simulink model "quad_1_ref_NN_ports_R2016a"  (R2016a)
settings: Solver=FixedStepAuto  SolverMode=SingleTasking  StartTime=0.0  StopTime=20  FixedStep=0.01  RelTol=1e-3
libraries: neural x416, simulink x2
(part 9 of 15)

== system quad_1_ref_NN_ports_R2016a/nn_2/Layer 3/Delays 1 ==
  "p{3}" : Inport  PortDimensions=30
      mask Display: e = 0.06;c1 = [120 230 180]/255;c2 = ([120 230 180]+0)/(256+128);c3 = ([120 230 180]+128)/(256+128);patch([0 1 1 0],[0 0 1 1],c1);patch([0 1 1 1-e 1-e 0+e],[0 0 1 1-e 0+e 0+e],c2);patch([0 0 1 1-e 0+e 0+e],[0 1 1 1-e 1-e 0+e],c3);plot([0 1 1 0 0],[0 0 1 1 0]);
  mux : Mux  Inputs=1
      mask Display: e = 0.06;c1 = [120 150 230]/255;c2 = ([120 150 230]+0)/383;c3 = ([120 150 230]+128)/383;patch([0 1 1 0],[0 0 1 1],c1);patch([0 1 1 1-e 1-e 0+e],[0 0 1 1-e 0+e 0+e],c2);patch([0 0 1 1-e 0+e 0+e],[0 1 1 1-e 1-e 0+e],c3);plot([0 1 1 0 0],[0 0 1 1 0]);disp('Mux')
  "pd{3,2}" : Outport
      mask Display: e = 0.06;c1 = [120 230 180]/255;c2 = ([120 230 180]+0)/(256+128);c3 = ([120 230 180]+128)/(256+128);patch([0 1 1 0],[0 0 1 1],c1);patch([0 1 1 1-e 1-e 0+e],[0 0 1 1-e 0+e 0+e],c2);patch([0 0 1 1-e 0+e 0+e],[0 1 1 1-e 1-e 0+e],c3);plot([0 1 1 0 0],[0 0 1 1 0]);
  wires:
  "p{3}"/1 -> mux/1
  mux/1 -> "pd{3,2}"/1

== system quad_1_ref_NN_ports_R2016a/nn_2/Layer 3/LW{3,2} ==
  "ad{3,2}" : Inport  PortDimensions=30
      mask Display: e = 0.06;c1 = [120 230 180]/255;c2 = ([120 230 180]+0)/(256+128);c3 = ([120 230 180]+128)/(256+128);patch([0 1 1 0],[0 0 1 1],c1);patch([0 1 1 1-e 1-e 0+e],[0 0 1 1-e 0+e 0+e],c2);patch([0 0 1 1-e 0+e 0+e],[0 1 1 1-e 1-e 0+e],c3);plot([0 1 1 0 0],[0 0 1 1 0]);
  "IW{3,2}(1,:)'" : Constant  Value=[-0.27926346020130399239178586867637932300567626953125;0.346606766393038834284112681416445411741733551025390625;-0.40463771690971828132177279258030466735363006591796875;0.374237250338739446675617728033103048801422119140625;0.253674479943673480963894917294965125620365142822265625;0.0770967057085971962937520629566279239952564239501953125;-0.202899235421085510910899074588087387382984161376953125;0.048789096197364538454177562698532710783183574676513671875;0.1969315529635952966014400544736417941749095916748046875;-0.22194913799231852369331363661331124603748321533203125;-0.10977738597411164367390057350348797626793384552001953125;-0.358002132240892556591660422782297246158123016357421875;-0.1503757586855622718768898948837886564433574676513671875;0.200219880617318768400991757516749203205108642578125;-0.123543856037150845406102916967938654124736785888671875;-0.0756290226239554608245185818304889835417270660400390625;0.09365695161798102963413015231708413921296596527099609375;-0.20471536813625856865428431774489581584930419921875;0.2120496832146524790463359977366053499281406402587890625;-0.372640774432040966512857949055614881217479705810546875;-0.0302653179057935893536690485916551551781594753265380859375;0.26262527413470404535900115661206655204296112060546875;0.135112314967465174664340565868769772350788116455078125;0.06986865315379715835053531236553681083023548126220703125;0.1380766631074236416854006392895826138556003570556640625;0.12643817431793713534915468699182383716106414794921875;-0.0841054694251663903514781850390136241912841796875;0.0107954259001523632244268213753457530401647090911865234375;-0.3098502314874116425613692626939155161380767822265625;-0.414602245804907398873950796769349835813045501708984375]
      mask Display: e = 0.06;c1 = [120 150 230]/255;c2 = ([120 150 230]+0)/383;c3 = ([120 150 230]+128)/383;patch([0 1 1 0],[0 0 1 1],c1);patch([0 1 1 1-e 1-e 0+e],[0 0 1 1-e 0+e 0+e],c2);patch([0 0 1 1-e 0+e 0+e],[0 1 1 1-e 1-e 0+e],c3);plot([0 1 1 0 0],[0 0 1 1 0]);disp('weights');
  "IW{3,2}(2,:)'" : Constant  Value=[-0.05747200023448355288291367060082848183810710906982421875;-0.0259577833702099060320112045019413926638662815093994140625;-0.0236994303769792295788487734853333677165210247039794921875;-0.031656006151221056932332231781401787884533405303955078125;0.02922803437695457862144365890344488434493541717529296875;-0.0138028700105828072697278230407391674816608428955078125;0.03581160208022715618625397837604396045207977294921875;0.112598189160304007483404120648629032075405120849609375;0.0278682772623776060794131836928499978967010974884033203125;0.01299548234236705922250987299548796727322041988372802734375;-0.0042449449882556132551680860842679976485669612884521484375;-0.0026716794761836083239858741222860771813429892063140869140625;-0.07927304809738729141077584472441230900585651397705078125;-0.0169222274978570695613822039149454212747514247894287109375;0.01453554486356052090345603033938459702767431735992431640625;0.0215353596980647384040441494335027527995407581329345703125;-0.04032680291918665227424156682900502346456050872802734375;-0.0759479482050604282061812000392819754779338836669921875;-0.006611013865375271227053932676653857924975454807281494140625;0.0031452949687314217704081631410417685401625931262969970703125;0.055297610322103320223963152102442109026014804840087890625;0.06198230119153878836524285134146339260041713714599609375;-0.0644313380485042885847946081412374041974544525146484375;-0.064363247549387880841464948389329947531223297119140625;-0.07785031888928649335124276831265888176858425140380859375;0.08416766991241975137683084540185518562793731689453125;0.0494813713765498708330170529734459705650806427001953125;-0.080233821303533348068270925068645738065242767333984375;-0.053953159457228984374754787722849869169294834136962890625;0.00844389404800993843835943408748789806850254535675048828125]
      mask Display: e = 0.06;c1 = [120 150 230]/255;c2 = ([120 150 230]+0)/383;c3 = ([120 150 230]+128)/383;patch([0 1 1 0],[0 0 1 1],c1);patch([0 1 1 1-e 1-e 0+e],[0 0 1 1-e 0+e 0+e],c2);patch([0 0 1 1-e 0+e 0+e],[0 1 1 1-e 1-e 0+e],c3);plot([0 1 1 0 0],[0 0 1 1 0]);disp('weights');
  "IW{3,2}(3,:)'" : Constant  Value=[-0.017218098925270992893832300296708126552402973175048828125;0.064559652034786141339139931005774997174739837646484375;-0.027977779266303494376533222975922399200499057769775390625;-0.01321248185154027567078660609922735602594912052154541015625;-0.0830621278421327657870421035113395191729068756103515625;-0.0010825688028150916471237241722747057792730629444122314453125;0.04702127339298324548710894532632664777338504791259765625;0.03579689634253153951437553814685088582336902618408203125;0.0722733893767697754828560618989286012947559356689453125;-0.001674565279581757305804590174602708430029451847076416015625;0.053646957375234116671691708688740618526935577392578125;0.07916322856407694008584741141021368093788623809814453125;-0.0129246026132422663079690750009831390343606472015380859375;0.059649020929645669986118861061186180450022220611572265625;-0.019698735030489515629437136112755979411303997039794921875;-0.052245577874222605407883435191251919604837894439697265625;-0.03210867066066773467536421549084479920566082000732421875;0.005740737672801155162816133525893746991641819477081298828125;-0.00965489046477303360094257556056618341244757175445556640625;-0.047030004358195674762921356659717275761067867279052734375;-0.03725889805072464533441944922742550261318683624267578125;0.052107784180737082291301476288936100900173187255859375;-0.060045653206628225861951619890533038415014743804931640625;-0.1206224460907344975257871055873692966997623443603515625;-0.00701652679878371487998123257057159207761287689208984375;0.1050073098366831880756677719546132721006870269775390625;-0.01056686890756637804689166415528234210796654224395751953125;-0.1311364635573339099128276075134635902941226959228515625;-0.054499355693794680755015491513404413126409053802490234375;0.05349236857790563848258358348175534047186374664306640625]
      mask Display: e = 0.06;c1 = [120 150 230]/255;c2 = ([120 150 230]+0)/383;c3 = ([120 150 230]+128)/383;patch([0 1 1 0],[0 0 1 1],c1);patch([0 1 1 1-e 1-e 0+e],[0 0 1 1-e 0+e 0+e],c2);patch([0 0 1 1-e 0+e 0+e],[0 1 1 1-e 1-e 0+e],c3);plot([0 1 1 0 0],[0 0 1 1 0]);disp('weights');
  Mux : Mux  Inputs=3
      mask Display: e = 0.06;c1 = [120 150 230]/255;c2 = ([120 150 230]+0)/383;c3 = ([120 150 230]+128)/383;patch([0 1 1 0],[0 0 1 1],c1);patch([0 1 1 1-e 1-e 0+e],[0 0 1 1-e 0+e 0+e],c2);patch([0 0 1 1-e 0+e 0+e],[0 1 1 1-e 1-e 0+e],c3);plot([0 1 1 0 0],[0 0 1 1 0]);disp('Mux');
  dotprod1 : neural/Weight Functions/dotprod
  dotprod2 : neural/Weight Functions/dotprod
  dotprod3 : neural/Weight Functions/dotprod
  "lz{3,2}" : Outport
      mask Display: e = 0.06;c1 = [120 230 180]/255;c2 = ([120 230 180]+0)/(256+128);c3 = ([120 230 180]+128)/(256+128);patch([0 1 1 0],[0 0 1 1],c1);patch([0 1 1 1-e 1-e 0+e],[0 0 1 1-e 0+e 0+e],c2);patch([0 0 1 1-e 0+e 0+e],[0 1 1 1-e 1-e 0+e],c3);plot([0 1 1 0 0],[0 0 1 1 0]);
  wires:
  "IW{3,2}(1,:)'"/1 -> dotprod1/1
  "ad{3,2}"/1 -> dotprod1/2, dotprod2/2, dotprod3/2
  dotprod1/1 -> Mux/1
  "IW{3,2}(2,:)'"/1 -> dotprod2/1
  dotprod2/1 -> Mux/2
  "IW{3,2}(3,:)'"/1 -> dotprod3/1
  dotprod3/1 -> Mux/3
  Mux/1 -> "lz{3,2}"/1

== system quad_1_ref_NN_ports_R2016a/nn_3_const/Layer 1/Delays 1 ==
  "p{1}" : Inport  PortDimensions=12
      mask Display: e = 0.06;c1 = [120 230 180]/255;c2 = ([120 230 180]+0)/(256+128);c3 = ([120 230 180]+128)/(256+128);patch([0 1 1 0],[0 0 1 1],c1);patch([0 1 1 1-e 1-e 0+e],[0 0 1 1-e 0+e 0+e],c2);patch([0 0 1 1-e 0+e 0+e],[0 1 1 1-e 1-e 0+e],c3);plot([0 1 1 0 0],[0 0 1 1 0]);
  mux : Mux  Inputs=1
      mask Display: e = 0.06;c1 = [120 150 230]/255;c2 = ([120 150 230]+0)/383;c3 = ([120 150 230]+128)/383;patch([0 1 1 0],[0 0 1 1],c1);patch([0 1 1 1-e 1-e 0+e],[0 0 1 1-e 0+e 0+e],c2);patch([0 0 1 1-e 0+e 0+e],[0 1 1 1-e 1-e 0+e],c3);plot([0 1 1 0 0],[0 0 1 1 0]);disp('Mux')
  "pd{1,1}" : Outport
      mask Display: e = 0.06;c1 = [120 230 180]/255;c2 = ([120 230 180]+0)/(256+128);c3 = ([120 230 180]+128)/(256+128);patch([0 1 1 0],[0 0 1 1],c1);patch([0 1 1 1-e 1-e 0+e],[0 0 1 1-e 0+e 0+e],c2);patch([0 0 1 1-e 0+e 0+e],[0 1 1 1-e 1-e 0+e],c3);plot([0 1 1 0 0],[0 0 1 1 0]);
  wires:
  "p{1}"/1 -> mux/1
  mux/1 -> "pd{1,1}"/1

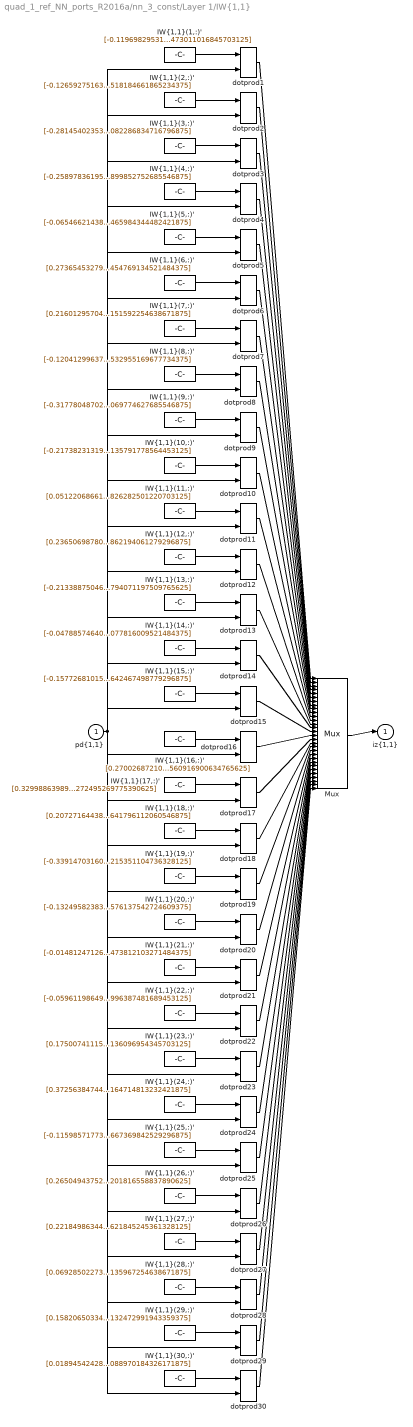
== system quad_1_ref_NN_ports_R2016a/nn_3_const/Layer 1/IW{1,1} ==
  "pd{1,1}" : Inport  PortDimensions=12
      mask Display: e = 0.06;c1 = [120 230 180]/255;c2 = ([120 230 180]+0)/(256+128);c3 = ([120 230 180]+128)/(256+128);patch([0 1 1 0],[0 0 1 1],c1);patch([0 1 1 1-e 1-e 0+e],[0 0 1 1-e 0+e 0+e],c2);patch([0 0 1 1-e 0+e 0+e],[0 1 1 1-e 1-e 0+e],c3);plot([0 1 1 0 0],[0 0 1 1 0]);
  "IW{1,1}(1,:)'" : Constant  Value=[-0.1196982953119827275401121369213797152042388916015625;-0.1289870733556734150315747911008656956255435943603515625;0.01486838419769767431766194221154364640824496746063232421875;-0.1972668416460273965729044221006915904581546783447265625;-0.1706947324630785356447404410573653876781463623046875;0.15527943735119176249526162791880778968334197998046875;0.280496872652939932546445334082818590104579925537109375;0.159230402032687179403325217208475805819034576416015625;-0.030182451792157276304617852247247355990111827850341796875;-0.09238192960821522969894203924923203885555267333984375;-0.09747367045827955156500621569648501463234424591064453125;0.1882049887453905168133161396326613612473011016845703125]
      mask Display: e = 0.06;c1 = [120 150 230]/255;c2 = ([120 150 230]+0)/383;c3 = ([120 150 230]+128)/383;patch([0 1 1 0],[0 0 1 1],c1);patch([0 1 1 1-e 1-e 0+e],[0 0 1 1-e 0+e 0+e],c2);patch([0 0 1 1-e 0+e 0+e],[0 1 1 1-e 1-e 0+e],c3);plot([0 1 1 0 0],[0 0 1 1 0]);disp('Weights');
  "IW{1,1}(10,:)'" : Constant  Value=[-0.2173823131999155500171383437191252596676349639892578125;-0.25150582247166453075948311379761435091495513916015625;-0.22407324408224360556829424240277148783206939697265625;-0.0178235762451871282419091357951401732861995697021484375;-0.0857934106951768471471808652495383284986019134521484375;0.19276250346259404810922433171072043478488922119140625;0.09913209349963171546082918439424247480928897857666015625;-0.0588047207570860652747768426706898026168346405029296875;-0.09416480925285675152025532952393405139446258544921875;0.1629371022116075373720178731673513539135456085205078125;-0.1852160572554303608061587738120579160749912261962890625;0.1669185592333850554069840654847212135791778564453125]
      mask Display: e = 0.06;c1 = [120 150 230]/255;c2 = ([120 150 230]+0)/383;c3 = ([120 150 230]+128)/383;patch([0 1 1 0],[0 0 1 1],c1);patch([0 1 1 1-e 1-e 0+e],[0 0 1 1-e 0+e 0+e],c2);patch([0 0 1 1-e 0+e 0+e],[0 1 1 1-e 1-e 0+e],c3);plot([0 1 1 0 0],[0 0 1 1 0]);disp('Weights');
  "IW{1,1}(11,:)'" : Constant  Value=[0.0512206866191046439329426220865570940077304840087890625;-0.1510948101597614223745580375179997645318508148193359375;-0.2129182130455107568867134659740258939564228057861328125;-0.342260556306487939703941947300336323678493499755859375;0.09978610256588016369505567126907408237457275390625;0.08653903693296537136259161115958704613149166107177734375;0.0034675135718981284389805797019334931974299252033233642578125;-0.178171083527447093874940264868200756609439849853515625;0.1926456653787382011788764657467254437506198883056640625;-0.2155749799301446556487604766516597010195255279541015625;-0.09451893403511162083940888578581507317721843719482421875;-0.04709443449216606236706894605958950705826282501220703125]
      mask Display: e = 0.06;c1 = [120 150 230]/255;c2 = ([120 150 230]+0)/383;c3 = ([120 150 230]+128)/383;patch([0 1 1 0],[0 0 1 1],c1);patch([0 1 1 1-e 1-e 0+e],[0 0 1 1-e 0+e 0+e],c2);patch([0 0 1 1-e 0+e 0+e],[0 1 1 1-e 1-e 0+e],c3);plot([0 1 1 0 0],[0 0 1 1 0]);disp('Weights');
  "IW{1,1}(12,:)'" : Constant  Value=[0.2365069878030960082160305546494782902300357818603515625;0.29432103747985538522158321939059533178806304931640625;0.2081499956215297764128280277873273007571697235107421875;0.25117398464888995857080544737982563674449920654296875;-0.2485034489625476961105476902957889251410961151123046875;0.158395104552063348268831077803042717278003692626953125;-0.1044569536603661419338351379337836988270282745361328125;-0.22613789129050088089201153707108460366725921630859375;-0.10573345075038453888538469982449896633625030517578125;0.02215455254487565250887115553268813528120517730712890625;0.027546109987116075557000982598765403963625431060791015625;-0.0492491638251608410126181070154416374862194061279296875]
      mask Display: e = 0.06;c1 = [120 150 230]/255;c2 = ([120 150 230]+0)/383;c3 = ([120 150 230]+128)/383;patch([0 1 1 0],[0 0 1 1],c1);patch([0 1 1 1-e 1-e 0+e],[0 0 1 1-e 0+e 0+e],c2);patch([0 0 1 1-e 0+e 0+e],[0 1 1 1-e 1-e 0+e],c3);plot([0 1 1 0 0],[0 0 1 1 0]);disp('Weights');
  "IW{1,1}(13,:)'" : Constant  Value=[-0.21338875046561300852232534452923573553562164306640625;-0.1340059789318859551077167679977719672024250030517578125;-0.1476616545504399746757684397380216978490352630615234375;0.214969424376130813225671545296791009604930877685546875;0.06644921596088482207420611302950419485569000244140625;-0.0117821724168989082348613095518885529600083827972412109375;-0.1872827624335566543134490302691119723021984100341796875;-0.082787703128192280388475410290993750095367431640625;0.1926407037939068256360286568451556377112865447998046875;0.277999477762065627661769440237549133598804473876953125;0.1379735123752584835532530860291444696485996246337890625;-0.1613026880844560528860398562756017781794071197509765625]
      mask Display: e = 0.06;c1 = [120 150 230]/255;c2 = ([120 150 230]+0)/383;c3 = ([120 150 230]+128)/383;patch([0 1 1 0],[0 0 1 1],c1);patch([0 1 1 1-e 1-e 0+e],[0 0 1 1-e 0+e 0+e],c2);patch([0 0 1 1-e 0+e 0+e],[0 1 1 1-e 1-e 0+e],c3);plot([0 1 1 0 0],[0 0 1 1 0]);disp('Weights');
  "IW{1,1}(14,:)'" : Constant  Value=[-0.04788574640253502601172641561788623221218585968017578125;0.15070670290952647984994428043137304484844207763671875;0.129709002988810606638026001746766269207000732421875;-0.07628835032242430036486524613792425952851772308349609375;-0.064693014780291324683503262349404394626617431640625;-0.120818118544549601978133068769238889217376708984375;-0.133195843769588317950791633847984485328197479248046875;-0.006931056317864360376279631026363858836703002452850341796875;0.07580874238176138479872179232188500463962554931640625;-0.1738726228089309266966466793746803887188434600830078125;0.08809580303368071130254435274764546193182468414306640625;-0.34741805583377372013131889616488479077816009521484375]
      mask Display: e = 0.06;c1 = [120 150 230]/255;c2 = ([120 150 230]+0)/383;c3 = ([120 150 230]+128)/383;patch([0 1 1 0],[0 0 1 1],c1);patch([0 1 1 1-e 1-e 0+e],[0 0 1 1-e 0+e 0+e],c2);patch([0 0 1 1-e 0+e 0+e],[0 1 1 1-e 1-e 0+e],c3);plot([0 1 1 0 0],[0 0 1 1 0]);disp('Weights');
  "IW{1,1}(15,:)'" : Constant  Value=[-0.1577268101593818083738796076431754045188426971435546875;-0.11256779664810658003748500277652055956423282623291015625;0.00802241259106954533730782230804834398441016674041748046875;0.19139711738853704137142131003201939165592193603515625;0.14056375245487162661817137632169760763645172119140625;0.169850393957305667580470753819099627435207366943359375;-0.162927276810809373852606540822307579219341278076171875;0.0411550400127098925384672156724263913929462432861328125;-0.09100914000223625510699321239371784031391143798828125;0.260212573300696636824369534224388189613819122314453125;0.2000730920156783276819822958714212290942668914794921875;0.211937407148370116072300106679904274642467498779296875]
      mask Display: e = 0.06;c1 = [120 150 230]/255;c2 = ([120 150 230]+0)/383;c3 = ([120 150 230]+128)/383;patch([0 1 1 0],[0 0 1 1],c1);patch([0 1 1 1-e 1-e 0+e],[0 0 1 1-e 0+e 0+e],c2);patch([0 0 1 1-e 0+e 0+e],[0 1 1 1-e 1-e 0+e],c3);plot([0 1 1 0 0],[0 0 1 1 0]);disp('Weights');
  "IW{1,1}(16,:)'" : Constant  Value=[0.27002687210488574010014417581260204315185546875;-0.04349468469703339501553074342155014164745807647705078125;0.1330845919116534492587788918172009289264678955078125;-0.182575685011664157197941449339850805699825286865234375;-0.10830309161015201635525073697863263078033924102783203125;0.239269603992316504115223096960107795894145965576171875;0.04760708347616089686216156451337155885994434356689453125;0.11252778570572473382238598560434184037148952484130859375;-0.1548024416375938516754473539549508132040500640869140625;-0.253057365838928294277110353505122475326061248779296875;-0.1250555668859235358691961437216377817094326019287109375;0.047842143321554821133734236582313315011560916900634765625]
      mask Display: e = 0.06;c1 = [120 150 230]/255;c2 = ([120 150 230]+0)/383;c3 = ([120 150 230]+128)/383;patch([0 1 1 0],[0 0 1 1],c1);patch([0 1 1 1-e 1-e 0+e],[0 0 1 1-e 0+e 0+e],c2);patch([0 0 1 1-e 0+e 0+e],[0 1 1 1-e 1-e 0+e],c3);plot([0 1 1 0 0],[0 0 1 1 0]);disp('Weights');
  "IW{1,1}(17,:)'" : Constant  Value=[0.3299886398943197018951423160615377128124237060546875;0.0808292241972947966832663269087788648903369903564453125;-0.02259926392819711082893263665027916431427001953125;0.054982407635770051690382587139538372866809368133544921875;-0.160980157363610765219874565445934422314167022705078125;0.1247636296345608908353597144014202058315277099609375;-0.035927420779184739141332016743035637773573398590087890625;0.08232447522588388910680379240147885866463184356689453125;-0.346576289182833063851063570837141014635562896728515625;-0.034377817283129170899957927076684427447617053985595703125;-0.2185372357072770943542394661562866531312465667724609375;-0.01525722862075677178916865983637762838043272495269775390625]
      mask Display: e = 0.06;c1 = [120 150 230]/255;c2 = ([120 150 230]+0)/383;c3 = ([120 150 230]+128)/383;patch([0 1 1 0],[0 0 1 1],c1);patch([0 1 1 1-e 1-e 0+e],[0 0 1 1-e 0+e 0+e],c2);patch([0 0 1 1-e 0+e 0+e],[0 1 1 1-e 1-e 0+e],c3);plot([0 1 1 0 0],[0 0 1 1 0]);disp('Weights');
  "IW{1,1}(18,:)'" : Constant  Value=[0.2072716443886149229047788367097382433712482452392578125;-0.158695591362616961195186604527407325804233551025390625;-0.194298743989455957592582535653491504490375518798828125;0.08089761317006245733285396681822021491825580596923828125;0.1275882176345632945668739921529777348041534423828125;0.166975404185521092426114364570821635425090789794921875;0.2179788041767063144771299221247318200767040252685546875;-0.2113613415917590943049475527004688046872615814208984375;-0.1680332296617765008850398089634836651384830474853515625;0.09479967011305796831255321421849657781422138214111328125;-0.10581935301708489394201251343474723398685455322265625;0.1349044775358076986293554000440053641796112060546875]
      mask Display: e = 0.06;c1 = [120 150 230]/255;c2 = ([120 150 230]+0)/383;c3 = ([120 150 230]+128)/383;patch([0 1 1 0],[0 0 1 1],c1);patch([0 1 1 1-e 1-e 0+e],[0 0 1 1-e 0+e 0+e],c2);patch([0 0 1 1-e 0+e 0+e],[0 1 1 1-e 1-e 0+e],c3);plot([0 1 1 0 0],[0 0 1 1 0]);disp('Weights');
  "IW{1,1}(19,:)'" : Constant  Value=[-0.33914703160923675984150804652017541229724884033203125;-0.10453048735648527711727950872955261729657649993896484375;-0.212564469375703168907421058975160121917724609375;0.10608477723513420887258007496711798012256622314453125;0.06988075897708780070960443708827369846403598785400390625;-0.028392761793704111850100701985866180621087551116943359375;0.036008968898993153062715322221265523694455623626708984375;-0.1601325327805253329049861577004776336252689361572265625;-0.016320432310186705482379920795210637152194976806640625;-0.22994571208807734752355145246838219463825225830078125;0.036023256587950823470745120857827714644372463226318359375;0.20727117665203309559984745646943338215351104736328125]
      mask Display: e = 0.06;c1 = [120 150 230]/255;c2 = ([120 150 230]+0)/383;c3 = ([120 150 230]+128)/383;patch([0 1 1 0],[0 0 1 1],c1);patch([0 1 1 1-e 1-e 0+e],[0 0 1 1-e 0+e 0+e],c2);patch([0 0 1 1-e 0+e 0+e],[0 1 1 1-e 1-e 0+e],c3);plot([0 1 1 0 0],[0 0 1 1 0]);disp('Weights');
  "IW{1,1}(2,:)'" : Constant  Value=[-0.1265927516381810391532525272850762121379375457763671875;-0.10406462981791535227227285531625966541469097137451171875;0.2148185548406552902722665976398275233805179595947265625;0.2371580895787383791439850710958126001060009002685546875;-0.2365432498183281662118560007002088241279125213623046875;0.05987656335314291144999998550702002830803394317626953125;0.0222476006243518854843532750464873970486223697662353515625;-0.11668078404641089862447955738389282487332820892333984375;-0.065758349599259913187410120372078381478786468505859375;-0.1329431588756458670896876128608710132539272308349609375;-0.1338080838789649507081236379235633648931980133056640625;0.1707220913756906932601253856773837469518184661865234375]
      mask Display: e = 0.06;c1 = [120 150 230]/255;c2 = ([120 150 230]+0)/383;c3 = ([120 150 230]+128)/383;patch([0 1 1 0],[0 0 1 1],c1);patch([0 1 1 1-e 1-e 0+e],[0 0 1 1-e 0+e 0+e],c2);patch([0 0 1 1-e 0+e 0+e],[0 1 1 1-e 1-e 0+e],c3);plot([0 1 1 0 0],[0 0 1 1 0]);disp('Weights');
  "IW{1,1}(20,:)'" : Constant  Value=[-0.13249582383027558307730942033231258392333984375;0.040030613773851704551010044497161288745701313018798828125;0.1702824726947762545847808723920024931430816650390625;-0.2408725064798178105984760577484848909080028533935546875;0.10623812004958511912011687172707752324640750885009765625;-0.139869975143498359582139300982817076146602630615234375;-0.1723200936692933227245561056406586430966854095458984375;-0.03984927795910563064207821071249782107770442962646484375;0.044199567930560519635196925491982256062328815460205078125;-0.2190396426762913628660811582449241541326045989990234375;0.1277829387419819051618929961477988399565219879150390625;0.170374810191310677165432707624859176576137542724609375]
      mask Display: e = 0.06;c1 = [120 150 230]/255;c2 = ([120 150 230]+0)/383;c3 = ([120 150 230]+128)/383;patch([0 1 1 0],[0 0 1 1],c1);patch([0 1 1 1-e 1-e 0+e],[0 0 1 1-e 0+e 0+e],c2);patch([0 0 1 1-e 0+e 0+e],[0 1 1 1-e 1-e 0+e],c3);plot([0 1 1 0 0],[0 0 1 1 0]);disp('Weights');
  "IW{1,1}(21,:)'" : Constant  Value=[-0.0148124712623549335821504513432955718599259853363037109375;-0.0311784914315909322812814252756652422249317169189453125;0.04522188239780784713151007281339843757450580596923828125;-0.2934434913415149281945559778250753879547119140625;0.171158930875923209757871745750890113413333892822265625;-0.1608476581751500933403775661645340733230113983154296875;-0.20675638704950161095297289648442529141902923583984375;0.348156303749445783513039032186497934162616729736328125;0.23679845860962200898569562923512421548366546630859375;0.223892726248125562005242272789473645389080047607421875;0.0289030250850557980657473677865709760226309299468994140625;-0.235499357660744423892396071096300147473812103271484375]
      mask Display: e = 0.06;c1 = [120 150 230]/255;c2 = ([120 150 230]+0)/383;c3 = ([120 150 230]+128)/383;patch([0 1 1 0],[0 0 1 1],c1);patch([0 1 1 1-e 1-e 0+e],[0 0 1 1-e 0+e 0+e],c2);patch([0 0 1 1-e 0+e 0+e],[0 1 1 1-e 1-e 0+e],c3);plot([0 1 1 0 0],[0 0 1 1 0]);disp('Weights');
  "IW{1,1}(22,:)'" : Constant  Value=[-0.059611986491373301910723370156119926832616329193115234375;0.2213751577076687737655191767771611921489238739013671875;0.1589485844453750740257191864657215774059295654296875;0.197716121842041570033643438364379107952117919921875;0.1514662645304741539487025647758855484426021575927734375;0.172775003422918349560433171063777990639209747314453125;0.203060971850576976738267376276780851185321807861328125;0.036534503618149305470552690167096443474292755126953125;0.077301466994075640482009248444228433072566986083984375;-0.1177192604996646074777544299649889580905437469482421875;0.12106019577847100532341784173695486970245838165283203125;-0.17993851102336766434319770269212312996387481689453125]
      mask Display: e = 0.06;c1 = [120 150 230]/255;c2 = ([120 150 230]+0)/383;c3 = ([120 150 230]+128)/383;patch([0 1 1 0],[0 0 1 1],c1);patch([0 1 1 1-e 1-e 0+e],[0 0 1 1-e 0+e 0+e],c2);patch([0 0 1 1-e 0+e 0+e],[0 1 1 1-e 1-e 0+e],c3);plot([0 1 1 0 0],[0 0 1 1 0]);disp('Weights');
  "IW{1,1}(23,:)'" : Constant  Value=[0.175007411157043712979231031567906029522418975830078125;-0.09330095053247415559649624583471450023353099822998046875;-0.215960552939064631683407924356288276612758636474609375;0.129472414805143209992621677884017117321491241455078125;-0.239940808198920496607797758770175278186798095703125;-0.069653398870320959446189590380527079105377197265625;-0.214353875622127210132106256423867307603359222412109375;0.0004286375228889800488400740885452933071064762771129608154296875;-0.0512173795049029878523327852235524915158748626708984375;0.11594052081714589785832458801451139152050018310546875;-0.1445651588249391716889391545919352211058139801025390625;-0.25233328001959531849962559135747142136096954345703125]
      mask Display: e = 0.06;c1 = [120 150 230]/255;c2 = ([120 150 230]+0)/383;c3 = ([120 150 230]+128)/383;patch([0 1 1 0],[0 0 1 1],c1);patch([0 1 1 1-e 1-e 0+e],[0 0 1 1-e 0+e 0+e],c2);patch([0 0 1 1-e 0+e 0+e],[0 1 1 1-e 1-e 0+e],c3);plot([0 1 1 0 0],[0 0 1 1 0]);disp('Weights');
  "IW{1,1}(24,:)'" : Constant  Value=[0.37256384744881809734096123065683059394359588623046875;-0.1432842251991764126461958994696033187210559844970703125;0.1377718344421794693932525888158124871551990509033203125;-0.589353589211446315943021545535884797573089599609375;-0.06178531294047295840954348022933118045330047607421875;-0.0154505347069833799678040264780065626837313175201416015625;0.1683078258323121578765579897662973962724208831787109375;-0.1664437272399152123458776486586430110037326812744140625;0.1873791777907282962711832396962563507258892059326171875;0.03288416218820687519919232499887584708631038665771484375;0.162765271872292782706637126466375775635242462158203125;-0.11285274050517050958841736019167001359164714813232421875]
      mask Display: e = 0.06;c1 = [120 150 230]/255;c2 = ([120 150 230]+0)/383;c3 = ([120 150 230]+128)/383;patch([0 1 1 0],[0 0 1 1],c1);patch([0 1 1 1-e 1-e 0+e],[0 0 1 1-e 0+e 0+e],c2);patch([0 0 1 1-e 0+e 0+e],[0 1 1 1-e 1-e 0+e],c3);plot([0 1 1 0 0],[0 0 1 1 0]);disp('Weights');
  "IW{1,1}(25,:)'" : Constant  Value=[-0.115985717734956583768735072226263582706451416015625;0.1493076208638430546482567251587170176208019256591796875;0.2002476867355400813597299247703631408512592315673828125;-0.26771207475659564156700298553914763033390045166015625;0.057630772409985257798137325835341471247375011444091796875;-0.1617184235669213432373680916498415172100067138671875;0.0887999943613410336329394567655981518328189849853515625;0.1870226133578477278884832912808633409440517425537109375;0.2072915270584706759482429561103344894945621490478515625;-0.1819923377068865255612450937405810691416263580322265625;-0.11884873510801842455553156696623773314058780670166015625;0.132748019518751536605094543119776062667369842529296875]
      mask Display: e = 0.06;c1 = [120 150 230]/255;c2 = ([120 150 230]+0)/383;c3 = ([120 150 230]+128)/383;patch([0 1 1 0],[0 0 1 1],c1);patch([0 1 1 1-e 1-e 0+e],[0 0 1 1-e 0+e 0+e],c2);patch([0 0 1 1-e 0+e 0+e],[0 1 1 1-e 1-e 0+e],c3);plot([0 1 1 0 0],[0 0 1 1 0]);disp('Weights');
  "IW{1,1}(26,:)'" : Constant  Value=[0.265049437520101960341634139695088379085063934326171875;-0.043127962986870327366517585687688551843166351318359375;0.06324231785530269600581476652223500423133373260498046875;-0.167145498219675392448380080168135464191436767578125;-0.10266957509710296359006775901434593833982944488525390625;0.07046395097403711227368461322839721105992794036865234375;-0.0400817962941015792921461979858577251434326171875;-0.120489126858635497985261508802068419754505157470703125;0.2112149275665802239387858207919634878635406494140625;0.1891994577758218387675270832914975471794605255126953125;-0.228634657789148099116260937080369330942630767822265625;-0.10414946107419044418751497005359851755201816558837890625]
      mask Display: e = 0.06;c1 = [120 150 230]/255;c2 = ([120 150 230]+0)/383;c3 = ([120 150 230]+128)/383;patch([0 1 1 0],[0 0 1 1],c1);patch([0 1 1 1-e 1-e 0+e],[0 0 1 1-e 0+e 0+e],c2);patch([0 0 1 1-e 0+e 0+e],[0 1 1 1-e 1-e 0+e],c3);plot([0 1 1 0 0],[0 0 1 1 0]);disp('Weights');
  "IW{1,1}(27,:)'" : Constant  Value=[0.2218498634465736751852915631388896144926548004150390625;-0.193833751064416082154906462164944969117641448974609375;0.177941926350075052543076026267954148352146148681640625;-0.189252378762839124082262287629419006407260894775390625;0.1302286515182972947979322952960501424968242645263671875;-0.08080312339151420053529051301666186191141605377197265625;0.190680986355462211978561981595703400671482086181640625;0.00784100937892250222926993075134305399842560291290283203125;-0.044533453815674979570093938718855497427284717559814453125;0.1226007069319831888076777204332756809890270233154296875;-0.143956039601102980807212361469282768666744232177734375;-0.1712952981268955898741523924400098621845245361328125]
      mask Display: e = 0.06;c1 = [120 150 230]/255;c2 = ([120 150 230]+0)/383;c3 = ([120 150 230]+128)/383;patch([0 1 1 0],[0 0 1 1],c1);patch([0 1 1 1-e 1-e 0+e],[0 0 1 1-e 0+e 0+e],c2);patch([0 0 1 1-e 0+e 0+e],[0 1 1 1-e 1-e 0+e],c3);plot([0 1 1 0 0],[0 0 1 1 0]);disp('Weights');
  "IW{1,1}(28,:)'" : Constant  Value=[0.069285022730961542958283416737685911357402801513671875;0.260500037412751350718309595322352834045886993408203125;0.258929936548664585416190675459802150726318359375;0.051862203376026420886812928756626206450164318084716796875;-0.268011929124568393234540053526870906352996826171875;-0.047632612230134978303919268682875554077327251434326171875;0.0213582840605084124663282096889815875329077243804931640625;-0.1722721696730589169277436667471192777156829833984375;-0.1408531121301170030424287915593595243990421295166015625;-0.061585673930256552843776063355107908137142658233642578125;0.21738059838316259320123435827554203569889068603515625;0.0870751102544260191518077363070915453135967254638671875]
      mask Display: e = 0.06;c1 = [120 150 230]/255;c2 = ([120 150 230]+0)/383;c3 = ([120 150 230]+128)/383;patch([0 1 1 0],[0 0 1 1],c1);patch([0 1 1 1-e 1-e 0+e],[0 0 1 1-e 0+e 0+e],c2);patch([0 0 1 1-e 0+e 0+e],[0 1 1 1-e 1-e 0+e],c3);plot([0 1 1 0 0],[0 0 1 1 0]);disp('Weights');
  "IW{1,1}(29,:)'" : Constant  Value=[0.158206503345123372650249393700505606830120086669921875;-0.1167115813229379350790537728244089521467685699462890625;-0.174624619944309167340890098785166628658771514892578125;0.118069241875576214084730963804759085178375244140625;0.0858192857803793673898695715251960791647434234619140625;0.1588419771976567751448072840503300540149211883544921875;0.11195652437048354832516139367726282216608524322509765625;-0.2078568334560400299171334381753695197403430938720703125;-0.1216025675984538645391097588799311779439449310302734375;0.1442203309680535061598760648848838172852993011474609375;-0.11457073589732448548605958649204694665968418121337890625;-0.2423468718021511703053505470961681567132472991943359375]
      mask Display: e = 0.06;c1 = [120 150 230]/255;c2 = ([120 150 230]+0)/383;c3 = ([120 150 230]+128)/383;patch([0 1 1 0],[0 0 1 1],c1);patch([0 1 1 1-e 1-e 0+e],[0 0 1 1-e 0+e 0+e],c2);patch([0 0 1 1-e 0+e 0+e],[0 1 1 1-e 1-e 0+e],c3);plot([0 1 1 0 0],[0 0 1 1 0]);disp('Weights');
  "IW{1,1}(3,:)'" : Constant  Value=[-0.28145402353184112431705443668761290609836578369140625;0.1260781948537200436444294382454245351254940032958984375;-0.141407770914534658412975431929226033389568328857421875;0.0823049572737721835125057623372413218021392822265625;-0.2050827811065634997955697826910181902348995208740234375;0.1652183450870099712393113122743670828640460968017578125;-0.147211741015504105067890350255765952169895172119140625;0.273411467720603928999167919755564071238040924072265625;0.1614958034400274800024277510601677931845188140869140625;-0.03454812947097267439300338764951447956264019012451171875;-0.05152166018603630825989370123352273367345333099365234375;-0.025257365527026613694072665339263039641082286834716796875]
      mask Display: e = 0.06;c1 = [120 150 230]/255;c2 = ([120 150 230]+0)/383;c3 = ([120 150 230]+128)/383;patch([0 1 1 0],[0 0 1 1],c1);patch([0 1 1 1-e 1-e 0+e],[0 0 1 1-e 0+e 0+e],c2);patch([0 0 1 1-e 0+e 0+e],[0 1 1 1-e 1-e 0+e],c3);plot([0 1 1 0 0],[0 0 1 1 0]);disp('Weights');
  "IW{1,1}(30,:)'" : Constant  Value=[0.018945424280687926665844855733666918240487575531005859375;0.1995715801428248614701743690602597780525684356689453125;0.12403009923170328632213710307041765190660953521728515625;-0.06135912715795650840266972636527498252689838409423828125;-0.032326994868567771046485859187669120728969573974609375;-0.1798706547556056245529276793604367412626743316650390625;-0.0160351695508717702332024401812304859049618244171142578125;-0.083546644247350254630646304576657712459564208984375;-0.1951457803110835664828215385568910278379917144775390625;-0.1691544971538902208951782313306466676294803619384765625;-0.2066097784601954867600426268836599774658679962158203125;-0.2325971246851534501853819847383419983088970184326171875]
      mask Display: e = 0.06;c1 = [120 150 230]/255;c2 = ([120 150 230]+0)/383;c3 = ([120 150 230]+128)/383;patch([0 1 1 0],[0 0 1 1],c1);patch([0 1 1 1-e 1-e 0+e],[0 0 1 1-e 0+e 0+e],c2);patch([0 0 1 1-e 0+e 0+e],[0 1 1 1-e 1-e 0+e],c3);plot([0 1 1 0 0],[0 0 1 1 0]);disp('Weights');
  "IW{1,1}(4,:)'" : Constant  Value=[-0.25897836195603141096199806270305998623371124267578125;-0.08773584389797840776825665898286388255655765533447265625;0.12015507045280286735344787985013681463897228240966796875;0.0361909909585266531539815559881390072405338287353515625;-0.2128536070269596847115423088325769640505313873291015625;0.1463695284926984918616454933726345188915729522705078125;0.30953078911182541066438034249586053192615509033203125;-0.2034985363635319621788966060194070450961589813232421875;-0.0885619727404492185218742861252394504845142364501953125;-0.05643587643771015571747540207070414908230304718017578125;-0.2063731608513614534938795941343414597213268280029296875;0.1133056984907023501119027741879108361899852752685546875]
      mask Display: e = 0.06;c1 = [120 150 230]/255;c2 = ([120 150 230]+0)/383;c3 = ([120 150 230]+128)/383;patch([0 1 1 0],[0 0 1 1],c1);patch([0 1 1 1-e 1-e 0+e],[0 0 1 1-e 0+e 0+e],c2);patch([0 0 1 1-e 0+e 0+e],[0 1 1 1-e 1-e 0+e],c3);plot([0 1 1 0 0],[0 0 1 1 0]);disp('Weights');
  "IW{1,1}(5,:)'" : Constant  Value=[-0.06546621438372472734368301416907343082129955291748046875;-0.1405605935952531637678220022280584089457988739013671875;-0.224987235141161701079681733972392976284027099609375;0.2334506280952731993583171288264566101133823394775390625;0.062248364259608467141671184208462364040315151214599609375;0.2226942814012638771625773870255216024816036224365234375;0.1768548726666858972311757725037750788033008575439453125;0.05880562753752312243893385357296210713684558868408203125;-0.002704041070264113881538303729712424683384597301483154296875;0.192654298910743093653508140050689689815044403076171875;-0.1480341744715330254411611576870200224220752716064453125;-0.002533840567329140140706567052575337584130465984344482421875]
      mask Display: e = 0.06;c1 = [120 150 230]/255;c2 = ([120 150 230]+0)/383;c3 = ([120 150 230]+128)/383;patch([0 1 1 0],[0 0 1 1],c1);patch([0 1 1 1-e 1-e 0+e],[0 0 1 1-e 0+e 0+e],c2);patch([0 0 1 1-e 0+e 0+e],[0 1 1 1-e 1-e 0+e],c3);plot([0 1 1 0 0],[0 0 1 1 0]);disp('Weights');
  "IW{1,1}(6,:)'" : Constant  Value=[0.27365453279568419109324395321891643106937408447265625;0.197726059436817258596619240051950328052043914794921875;-0.0072955368385953338339344753649129415862262248992919921875;-0.2061881454872402097411310251118266023695468902587890625;-0.038749288167260032000882574720890261232852935791015625;-0.05547171267713270348398424403058015741407871246337890625;0.1679057257558425886312392094623646698892116546630859375;-0.0414595752067529466078354971614317037165164947509765625;0.178530451392176214842066883647930808365345001220703125;-0.03640738667940700279412880036034039221704006195068359375;0.2285938841786141761946993256060522980988025665283203125;-0.2424753635010881980260677437399863265454769134521484375]
      mask Display: e = 0.06;c1 = [120 150 230]/255;c2 = ([120 150 230]+0)/383;c3 = ([120 150 230]+128)/383;patch([0 1 1 0],[0 0 1 1],c1);patch([0 1 1 1-e 1-e 0+e],[0 0 1 1-e 0+e 0+e],c2);patch([0 0 1 1-e 0+e 0+e],[0 1 1 1-e 1-e 0+e],c3);plot([0 1 1 0 0],[0 0 1 1 0]);disp('Weights');
  "IW{1,1}(7,:)'" : Constant  Value=[0.2160129570444971058851280076851253397762775421142578125;0.097861179279611965053931044167256914079189300537109375;-0.229475954607031129572902727886685170233249664306640625;0.1812519622862836798926622350336401723325252532958984375;0.049553276304841402388756677055425825528800487518310546875;0.1867743365476895733845452696186839602887630462646484375;0.1409861299478845919619374171816161833703517913818359375;-0.048506754115844319397155004480737261474132537841796875;0.098665510640499609618103704633540473878383636474609375;-0.2369588138670304100497077115505817346274852752685546875;-0.159457335688088452929633831445244140923023223876953125;-0.2485815610364112415719972659644554369151592254638671875]
      mask Display: e = 0.06;c1 = [120 150 230]/255;c2 = ([120 150 230]+0)/383;c3 = ([120 150 230]+128)/383;patch([0 1 1 0],[0 0 1 1],c1);patch([0 1 1 1-e 1-e 0+e],[0 0 1 1-e 0+e 0+e],c2);patch([0 0 1 1-e 0+e 0+e],[0 1 1 1-e 1-e 0+e],c3);plot([0 1 1 0 0],[0 0 1 1 0]);disp('Weights');
  "IW{1,1}(8,:)'" : Constant  Value=[-0.12041299637619475026983906218447373248636722564697265625;-0.1962096873375609173972833332300069741904735565185546875;-0.19620131729035572565322809168719686567783355712890625;-0.27612644098689764771137333809747360646724700927734375;0.238387583207555653341813695078599266707897186279296875;-0.1594228760434201197515591275077895261347293853759765625;-0.14367926659173868575436472383444197475910186767578125;-0.005613168386785973018593409733512089587748050689697265625;0.2237440678436710406185028432446415536105632781982421875;-0.137269406742873745219668535355594940483570098876953125;-0.081922920100877372195924408515566028654575347900390625;-0.11978169095285561007724339788182987831532955169677734375]
      mask Display: e = 0.06;c1 = [120 150 230]/255;c2 = ([120 150 230]+0)/383;c3 = ([120 150 230]+128)/383;patch([0 1 1 0],[0 0 1 1],c1);patch([0 1 1 1-e 1-e 0+e],[0 0 1 1-e 0+e 0+e],c2);patch([0 0 1 1-e 0+e 0+e],[0 1 1 1-e 1-e 0+e],c3);plot([0 1 1 0 0],[0 0 1 1 0]);disp('Weights');
  "IW{1,1}(9,:)'" : Constant  Value=[-0.31778048702674066561257859575562179088592529296875;-0.331955299976685769269835191153106279671192169189453125;-0.160727837188179567551316040407982654869556427001953125;0.1310478788871549393757476309474441222846508026123046875;-0.1511889025791886831395771650932147167623043060302734375;0.10052959214114846886456433594503323547542095184326171875;0.325633087451002223300378091153106652200222015380859375;-0.138914828189722616702539426114526577293872833251953125;0.01835917903745178103580570905251079238951206207275390625;0.07985474121231124489117547682326403446495532989501953125;-0.01218709622126272658360068845695423078723251819610595703125;0.14152448302326614548718453079345636069774627685546875]
      mask Display: e = 0.06;c1 = [120 150 230]/255;c2 = ([120 150 230]+0)/383;c3 = ([120 150 230]+128)/383;patch([0 1 1 0],[0 0 1 1],c1);patch([0 1 1 1-e 1-e 0+e],[0 0 1 1-e 0+e 0+e],c2);patch([0 0 1 1-e 0+e 0+e],[0 1 1 1-e 1-e 0+e],c3);plot([0 1 1 0 0],[0 0 1 1 0]);disp('Weights');
  Mux : Mux  Inputs=30
      mask Display: e = 0.06;c1 = [120 150 230]/255;c2 = ([120 150 230]+0)/383;c3 = ([120 150 230]+128)/383;patch([0 1 1 0],[0 0 1 1],c1);patch([0 1 1 1-e 1-e 0+e],[0 0 1 1-e 0+e 0+e],c2);patch([0 0 1 1-e 0+e 0+e],[0 1 1 1-e 1-e 0+e],c3);plot([0 1 1 0 0],[0 0 1 1 0]);disp('Mux');
  dotprod{1..30} (30 alike) : neural/Weight Functions/dotprod
  "iz{1,1}" : Outport
      mask Display: e = 0.06;c1 = [120 230 180]/255;c2 = ([120 230 180]+0)/(256+128);c3 = ([120 230 180]+128)/(256+128);patch([0 1 1 0],[0 0 1 1],c1);patch([0 1 1 1-e 1-e 0+e],[0 0 1 1-e 0+e 0+e],c2);patch([0 0 1 1-e 0+e 0+e],[0 1 1 1-e 1-e 0+e],c3);plot([0 1 1 0 0],[0 0 1 1 0]);
  wires:
  "IW{1,1}(1,:)'"/1 -> dotprod1/1
  "pd{1,1}"/1 -> dotprod1/2, dotprod2/2, dotprod3/2, dotprod4/2, dotprod5/2, dotprod6/2, dotprod7/2, dotprod8/2, dotprod9/2, dotprod10/2, dotprod11/2, dotprod12/2, dotprod13/2, dotprod14/2, dotprod15/2, dotprod16/2, dotprod17/2, dotprod18/2, dotprod19/2, dotprod20/2, dotprod21/2, dotprod22/2, dotprod23/2, dotprod24/2, dotprod25/2, dotprod26/2, dotprod27/2, dotprod28/2, dotprod29/2, dotprod30/2
  dotprod1/1 -> Mux/1
  "IW{1,1}(2,:)'"/1 -> dotprod2/1
  dotprod2/1 -> Mux/2
  "IW{1,1}(3,:)'"/1 -> dotprod3/1
  dotprod3/1 -> Mux/3
  "IW{1,1}(4,:)'"/1 -> dotprod4/1
  dotprod4/1 -> Mux/4
  "IW{1,1}(5,:)'"/1 -> dotprod5/1
  dotprod5/1 -> Mux/5
  "IW{1,1}(6,:)'"/1 -> dotprod6/1
  dotprod6/1 -> Mux/6
  "IW{1,1}(7,:)'"/1 -> dotprod7/1
  dotprod7/1 -> Mux/7
  "IW{1,1}(8,:)'"/1 -> dotprod8/1
  dotprod8/1 -> Mux/8
  "IW{1,1}(9,:)'"/1 -> dotprod9/1
  dotprod9/1 -> Mux/9
  "IW{1,1}(10,:)'"/1 -> dotprod10/1
  dotprod10/1 -> Mux/10
  "IW{1,1}(11,:)'"/1 -> dotprod11/1
  dotprod11/1 -> Mux/11
  "IW{1,1}(12,:)'"/1 -> dotprod12/1
  dotprod12/1 -> Mux/12
  "IW{1,1}(13,:)'"/1 -> dotprod13/1
  dotprod13/1 -> Mux/13
  "IW{1,1}(14,:)'"/1 -> dotprod14/1
  dotprod14/1 -> Mux/14
  "IW{1,1}(15,:)'"/1 -> dotprod15/1
  dotprod15/1 -> Mux/15
  "IW{1,1}(16,:)'"/1 -> dotprod16/1
  dotprod16/1 -> Mux/16
  "IW{1,1}(17,:)'"/1 -> dotprod17/1
  dotprod17/1 -> Mux/17
  "IW{1,1}(18,:)'"/1 -> dotprod18/1
  dotprod18/1 -> Mux/18
  "IW{1,1}(19,:)'"/1 -> dotprod19/1
  dotprod19/1 -> Mux/19
  "IW{1,1}(20,:)'"/1 -> dotprod20/1
  dotprod20/1 -> Mux/20
  "IW{1,1}(21,:)'"/1 -> dotprod21/1
  dotprod21/1 -> Mux/21
  "IW{1,1}(22,:)'"/1 -> dotprod22/1
  dotprod22/1 -> Mux/22
  "IW{1,1}(23,:)'"/1 -> dotprod23/1
  dotprod23/1 -> Mux/23
  "IW{1,1}(24,:)'"/1 -> dotprod24/1
  dotprod24/1 -> Mux/24
  "IW{1,1}(25,:)'"/1 -> dotprod25/1
  dotprod25/1 -> Mux/25
  "IW{1,1}(26,:)'"/1 -> dotprod26/1
  dotprod26/1 -> Mux/26
  "IW{1,1}(27,:)'"/1 -> dotprod27/1
  dotprod27/1 -> Mux/27
  "IW{1,1}(28,:)'"/1 -> dotprod28/1
  dotprod28/1 -> Mux/28
  "IW{1,1}(29,:)'"/1 -> dotprod29/1
  dotprod29/1 -> Mux/29
  "IW{1,1}(30,:)'"/1 -> dotprod30/1
  dotprod30/1 -> Mux/30
  Mux/1 -> "iz{1,1}"/1

== system quad_1_ref_NN_ports_R2016a/nn_3_const/Layer 2/Delays 1 ==
  "p{2}" : Inport  PortDimensions=30
      mask Display: e = 0.06;c1 = [120 230 180]/255;c2 = ([120 230 180]+0)/(256+128);c3 = ([120 230 180]+128)/(256+128);patch([0 1 1 0],[0 0 1 1],c1);patch([0 1 1 1-e 1-e 0+e],[0 0 1 1-e 0+e 0+e],c2);patch([0 0 1 1-e 0+e 0+e],[0 1 1 1-e 1-e 0+e],c3);plot([0 1 1 0 0],[0 0 1 1 0]);
  mux : Mux  Inputs=1
      mask Display: e = 0.06;c1 = [120 150 230]/255;c2 = ([120 150 230]+0)/383;c3 = ([120 150 230]+128)/383;patch([0 1 1 0],[0 0 1 1],c1);patch([0 1 1 1-e 1-e 0+e],[0 0 1 1-e 0+e 0+e],c2);patch([0 0 1 1-e 0+e 0+e],[0 1 1 1-e 1-e 0+e],c3);plot([0 1 1 0 0],[0 0 1 1 0]);disp('Mux')
  "pd{2,1}" : Outport
      mask Display: e = 0.06;c1 = [120 230 180]/255;c2 = ([120 230 180]+0)/(256+128);c3 = ([120 230 180]+128)/(256+128);patch([0 1 1 0],[0 0 1 1],c1);patch([0 1 1 1-e 1-e 0+e],[0 0 1 1-e 0+e 0+e],c2);patch([0 0 1 1-e 0+e 0+e],[0 1 1 1-e 1-e 0+e],c3);plot([0 1 1 0 0],[0 0 1 1 0]);
  wires:
  "p{2}"/1 -> mux/1
  mux/1 -> "pd{2,1}"/1
